simulink model "Torre"  (R2023a)
settings: Solver=VariableStepAuto  StartTime=0.0  StopTime=10  RelTol=1e-3
values from neighbouring files (symbols this model uses):
  a = 5.68    [setup.m]    (also in setup_simple.m)
  B = 14.32    [setup.m]    (also in setup_simple.m)
  D = 8.7775    [setup.m]    (also in setup_simple.m)
  L = 7.3916    [setup.m]    (also in setup_simple.m)
  Lf = 13.3973    [setup.m]    (also in setup_simple.m)
  M = 5.80    (= 5.8)    [setup.m]    (also in setup_simple.m)
  Mb = 31.11    [setup.m]    (also in setup_simple.m)
  Md = 13.07    [setup.m]    (also in setup_simple.m)
  V = 6.4677    [setup.m]    (also in setup_simple.m)
  Vf = 9.7015    [setup.m]    (also in setup_simple.m)
  XF = 0.26095    [setup.m]    (also in setup_simple.m)
  YF = 0.66728    [setup.m]    (also in setup_simple.m)
libraries: slpidlib x2
settings Model: Creator=11106979966  LastModifiedBy=pedro
settings SolverCC: ZeroCrossAlgorithm=Adaptive  AlgebraicLoopSolver=TrustRegion
settings DataIOCC: ReturnWorkspaceOutputs=off
settings DebuggingCC: IgnoredZcDiagnostic=none  UnconnectedInputMsg=warning  UnconnectedOutputMsg=warning  UnconnectedLineMsg=warning  ArithmeticOperatorsInVariantConditions=warning
settings ModelReferenceCC: EnableRefExpFcnMdlSchedulingChecks=on
settings SFSimCC: SimUseLocalCustomCode=off  CustomCodeUndefinedFunction=UseInterfaceOnly
settings RTWCC: RTWUseLocalCustomCode=off
settings CodeAppCC: StateflowObjectComments=on

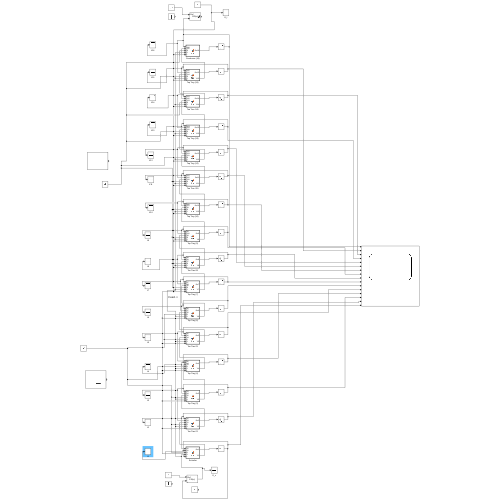
[thumbnail: Simulink's stored preview of the top-level diagram]
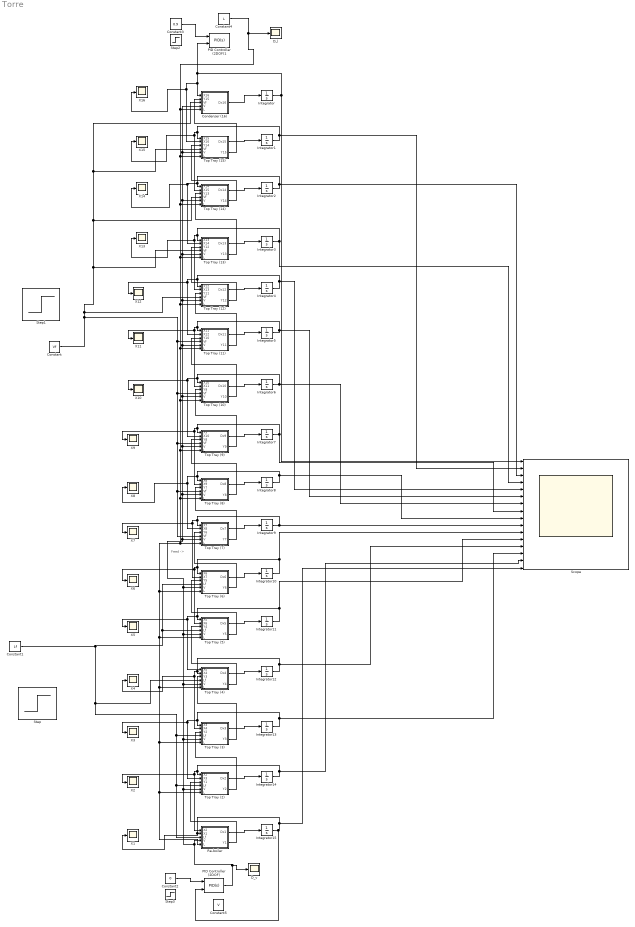
== system Torre ==
  note: Feed ->
  "Condenser (16) " : MATLAB Function  TreatAsAtomicUnit=on
  Constant : Constant  Value=Vf
  Constant1 : Constant  Value=Lf
  Constant2 : Constant  Value=0
  Constant3 : Constant  Value=0.9
  Constant4 : Constant  Value=L
  Constant5 : Constant  Value=V
  D_l : Scope
  D_v : Scope
  Integrator{,1..15} (16 alike) : Integrator  LimitOutput=on  UpperSaturationLimit=1  LowerSaturationLimit=0
  PID Controller (2DOF) : slpidlib/PID Controller (2DOF)  Controller=PID  Form=Parallel  TimeDomain=Continuous-time  UseExternalTs=off  SampleTime=-1  IntegratorMethod=Forward Euler  FilterMethod=Forward Euler  ControllerParametersSource=internal  P=-10000  I=0  UseKiTs=off  D=0  N=100  UseFilter=on  b=1  c=1  TunerSelectOption=Transfer Function Based (PID Tuner App)  InitialConditionSource=internal  InitialConditionForIntegrator=0  InitialConditionForFilter=0  DifferentiatorICPrevScaledInput=0  ExternalReset=none  TrackingMode=off  Kt=1  LimitOutput=off  SatLimitsSource=internal  UpperSaturationLimit=inf  LowerSaturationLimit=-inf  LinearizeAsGain=on  AntiWindupMode=none  Kb=1  LimitIntegrator=off  UpperIntegratorSaturationLimit=inf  LowerIntegratorSaturationLimit=-inf  POutMin=[]  POutMax=[]  IOutMin=[]  IOutMax=[]  DOutMin=[]  DOutMax=[]  NOutMin=[]  NOutMax=[]  bOutMin=[]  bOutMax=[]  cOutMin=[]  cOutMax=[]  SumOutMin=[]  SumOutMax=[]  SaturationOutMin=[]  SaturationOutMax=[]  PParamMin=[]  PParamMax=[]  IParamMin=[]  IParamMax=[]  DParamMin=[]  DParamMax=[]  NParamMin=[]  NParamMax=[]  bParamMin=[]  bParamMax=[]  cParamMin=[]  cParamMax=[]  KbParamMin=[]  KbParamMax=[]  KtParamMin=[]  KtParamMax=[]  KbOutMin=[]  KbOutMax=[]  KtOutMin=[]  KtOutMax=[]  IntegratorOutMin=[]  IntegratorOutMax=[]  FilterOutMin=[]  FilterOutMax=[]  SumI1OutMin=[]  SumI1OutMax=[]  SumI2OutMin=[]  SumI2OutMax=[]  SumI3OutMin=[]  SumI3OutMax=[]  SumI4OutMin=[]  SumI4OutMax=[]  SumDOutMin=[]  SumDOutMax=[]  Sum1OutMin=[]  Sum1OutMax=[]  Sum2OutMin=[]  Sum2OutMax=[]  Sum3OutMin=[]  Sum3OutMax=[]  DifferentiatorOutMin=[]  DifferentiatorOutMax=[]  FilterDiffOutCoefMin=[]  FilterDiffOutCoefMax=[]  ReciprocalOutMin=[]  ReciprocalOutMax=[]  SumDenOutMin=[]  SumDenOutMax=[]  SumNumOutMin=[]  SumNumOutMax=[]  DivideOutMin=[]  DivideOutMax=[]  UdiffTsProdOutMin=[]  UdiffTsProdOutMax=[]  NTsProdOutMin=[]  NTsProdOutMax=[]  UintegralTsProdOutMin=[]  UintegralTsProdOutMax=[]  UngainTsProdOutMin=[]  UngainTsProdOutMax=[]  ClampingZeroOutDataTypeStr=Inherit: Inherit via back propagation  ClampingZeroOutMin=[]  ClampingZeroOutMax=[]  FilterDenConstantOutDataTypeStr=Inherit: Inherit via back propagation  FilterDenConstantOutMin=[]  FilterDenConstantOutMax=[]  PCopyOutDataTypeStr=Inherit: Inherit via back propagation  PCopyOutMin=[]  PCopyOutMax=[]  NCopyOutDataTypeStr=Inherit: Inherit via back propagation  NCopyOutMin=[]  NCopyOutMax=[]  IntegratorContinuousStateAttributes=''  IntegratorStateMustResolveToSignalObject=off  IntegratorRTWStateStorageClass=Auto  FilterContinuousStateAttributes=''  FilterStateMustResolveToSignalObject=off  FilterRTWStateStorageClass=Auto  ParallelPVariant=InternalParameters  IdealPVariant=Disabled  IVariant=InternalParameters  DVariant=InternalParameters  bVariant=InternalParameters  cVariant=InternalParameters  IntegratorVariant=Continuous  SatVariant=Disabled  AWVariant=Passthrough  PCopyVariant=Disabled  TRVariant=Disabled  FdbkBlocksVariant=Forward  IdealPFdbkVariant=Disabled  SatFdbkVariant=Disabled  DerivativeFilterVariant=ContFilter  NVariant=InternalParameters  NCopyVariant=Disabled  FilterICVariant=InternalICsFilter  IntegratorICVariant=InternalICs  ExternalResetVariant=Disabled  TRSumVariant=Passthrough  SumFdbkVariant=Disabled  SumVariant=Sum_PID  TsampFilterVariant=InternalTs  TsampNgainVariant=Passthrough  TsampIntegralVariant=Disabled_SignalSpec  ExternalSaturationOutDataTypeStr=Inherit: Same as second input
  PID Controller (2DOF)1 : slpidlib/PID Controller (2DOF)  Controller=PID  Form=Parallel  TimeDomain=Continuous-time  UseExternalTs=off  SampleTime=-1  IntegratorMethod=Forward Euler  FilterMethod=Forward Euler  ControllerParametersSource=internal  P=-1000  I=0  UseKiTs=off  D=0.7  N=100  UseFilter=on  b=1  c=1  TunerSelectOption=Transfer Function Based (PID Tuner App)  InitialConditionSource=internal  InitialConditionForIntegrator=0  InitialConditionForFilter=0  DifferentiatorICPrevScaledInput=0  ExternalReset=none  TrackingMode=off  Kt=1  LimitOutput=on  SatLimitsSource=internal  UpperSaturationLimit=inf  LowerSaturationLimit=0  LinearizeAsGain=on  AntiWindupMode=none  Kb=1  LimitIntegrator=off  UpperIntegratorSaturationLimit=inf  LowerIntegratorSaturationLimit=-inf  POutMin=[]  POutMax=[]  IOutMin=[]  IOutMax=[]  DOutMin=[]  DOutMax=[]  NOutMin=[]  NOutMax=[]  bOutMin=[]  bOutMax=[]  cOutMin=[]  cOutMax=[]  SumOutMin=[]  SumOutMax=[]  SaturationOutMin=[]  SaturationOutMax=[]  PParamMin=[]  PParamMax=[]  IParamMin=[]  IParamMax=[]  DParamMin=[]  DParamMax=[]  NParamMin=[]  NParamMax=[]  bParamMin=[]  bParamMax=[]  cParamMin=[]  cParamMax=[]  KbParamMin=[]  KbParamMax=[]  KtParamMin=[]  KtParamMax=[]  KbOutMin=[]  KbOutMax=[]  KtOutMin=[]  KtOutMax=[]  IntegratorOutMin=[]  IntegratorOutMax=[]  FilterOutMin=[]  FilterOutMax=[]  SumI1OutMin=[]  SumI1OutMax=[]  SumI2OutMin=[]  SumI2OutMax=[]  SumI3OutMin=[]  SumI3OutMax=[]  SumI4OutMin=[]  SumI4OutMax=[]  SumDOutMin=[]  SumDOutMax=[]  Sum1OutMin=[]  Sum1OutMax=[]  Sum2OutMin=[]  Sum2OutMax=[]  Sum3OutMin=[]  Sum3OutMax=[]  DifferentiatorOutMin=[]  DifferentiatorOutMax=[]  FilterDiffOutCoefMin=[]  FilterDiffOutCoefMax=[]  ReciprocalOutMin=[]  ReciprocalOutMax=[]  SumDenOutMin=[]  SumDenOutMax=[]  SumNumOutMin=[]  SumNumOutMax=[]  DivideOutMin=[]  DivideOutMax=[]  UdiffTsProdOutMin=[]  UdiffTsProdOutMax=[]  NTsProdOutMin=[]  NTsProdOutMax=[]  UintegralTsProdOutMin=[]  UintegralTsProdOutMax=[]  UngainTsProdOutMin=[]  UngainTsProdOutMax=[]  ClampingZeroOutDataTypeStr=Inherit: Inherit via back propagation  ClampingZeroOutMin=[]  ClampingZeroOutMax=[]  FilterDenConstantOutDataTypeStr=Inherit: Inherit via back propagation  FilterDenConstantOutMin=[]  FilterDenConstantOutMax=[]  PCopyOutDataTypeStr=Inherit: Inherit via back propagation  PCopyOutMin=[]  PCopyOutMax=[]  NCopyOutDataTypeStr=Inherit: Inherit via back propagation  NCopyOutMin=[]  NCopyOutMax=[]  IntegratorContinuousStateAttributes=''  IntegratorStateMustResolveToSignalObject=off  IntegratorRTWStateStorageClass=Auto  FilterContinuousStateAttributes=''  FilterStateMustResolveToSignalObject=off  FilterRTWStateStorageClass=Auto  ParallelPVariant=InternalParameters  IdealPVariant=Disabled  IVariant=InternalParameters  DVariant=InternalParameters  bVariant=InternalParameters  cVariant=InternalParameters  IntegratorVariant=Continuous  SatVariant=Enabled  AWVariant=Passthrough  PCopyVariant=Disabled  TRVariant=Disabled  FdbkBlocksVariant=Forward  IdealPFdbkVariant=Disabled  SatFdbkVariant=Disabled  DerivativeFilterVariant=ContFilter  NVariant=InternalParameters  NCopyVariant=Disabled  FilterICVariant=InternalICsFilter  IntegratorICVariant=InternalICs  ExternalResetVariant=Disabled  TRSumVariant=Passthrough  SumFdbkVariant=Disabled  SumVariant=Sum_PID  TsampFilterVariant=InternalTs  TsampNgainVariant=Passthrough  TsampIntegralVariant=Disabled_SignalSpec  ExternalSaturationOutDataTypeStr=Inherit: Same as second input
  Re-boiler : MATLAB Function  TreatAsAtomicUnit=on
  Scope : Scope  NumInputPorts=16
  Step : Step  Time=150  Before=13.3973  After=8.5  SampleTime=0
  Step1 : Step  Time=150  Before=9.7015  After=15.6258  SampleTime=0
  Step2 : Step  Time=20  Before=0.8  SampleTime=0
  Step3 : Step  Time=50  After=0.1  SampleTime=0
  Top Tray (10) : MATLAB Function  TreatAsAtomicUnit=on
  Top Tray (11) : MATLAB Function  TreatAsAtomicUnit=on
  Top Tray (12) : MATLAB Function  TreatAsAtomicUnit=on
  Top Tray (13) : MATLAB Function  TreatAsAtomicUnit=on
  Top Tray (14) : MATLAB Function  TreatAsAtomicUnit=on
  Top Tray (15) : MATLAB Function  TreatAsAtomicUnit=on
  Top Tray (2) : MATLAB Function  TreatAsAtomicUnit=on
  Top Tray (3) : MATLAB Function  TreatAsAtomicUnit=on
  Top Tray (4) : MATLAB Function  TreatAsAtomicUnit=on
  Top Tray (5) : MATLAB Function  TreatAsAtomicUnit=on
  Top Tray (6) : MATLAB Function  TreatAsAtomicUnit=on
  Top Tray (7) : MATLAB Function  TreatAsAtomicUnit=on
  Top Tray (8) : MATLAB Function  TreatAsAtomicUnit=on
  Top Tray (9) : MATLAB Function  TreatAsAtomicUnit=on
  X{1..12} (12 alike) : Scope
  "X13 " : Scope
  "X14 " : Scope
  "X15 " : Scope
  "X16 " : Scope
  wires:
  "Condenser (16) "/1(Dx16) -> Integrator/1
  Integrator/1 -> PID Controller (2DOF)1/2, "X16 "/1, Top Tray (15)/2(X16), "Condenser (16) "/1(X16), Scope/1
  Top Tray (15)/1(Dx15) -> Integrator1/1
  Top Tray (14)/1(Dx14) -> Integrator2/1
  Integrator2/1 -> "X14 "/1, Top Tray (13)/2(X14), Top Tray (14)/1(X14), Scope/3
  Top Tray (13)/1(Dx13) -> Integrator3/1
  Integrator3/1 -> "X13 "/1, Top Tray (12)/2(X13), Top Tray (13)/1(X13), Scope/4
  Integrator4/1 -> Scope/5, X12/1, Top Tray (11)/2(X12), Top Tray (12)/1(X12)
  Top Tray (12)/1(Dx12) -> Integrator4/1
  Integrator5/1 -> X11/1, Top Tray (10)/2(X11), Top Tray (11)/1(X11), Scope/6
  Top Tray (11)/1(Dx11) -> Integrator5/1
  Integrator6/1 -> Top Tray (9)/2(X10), X10/1, Top Tray (10)/1(X10), Scope/7
  Top Tray (10)/1(Dx10) -> Integrator6/1
  Top Tray (9)/1(Dx9) -> Integrator7/1
  Integrator7/1 -> X9/1, Top Tray (8)/2(X9), Top Tray (9)/1(X9), Scope/8
  Integrator8/1 -> Scope/9, X8/1, Top Tray (7)/2(X8), Top Tray (8)/1(X8)
  Top Tray (8)/1(Dx8) -> Integrator8/1
  Integrator9/1 -> X7/1, Top Tray (6)/2(X7), Top Tray (7)/1(X7), Scope/10
  Top Tray (7)/1(Dx7) -> Integrator9/1
  Top Tray (6)/1(Dx6) -> Integrator10/1
  Top Tray (5)/1(Dx5) -> Integrator11/1
  Top Tray (4)/1(Dx4) -> Integrator12/1
  Integrator12/1 -> Scope/13, X4/1, Top Tray (3)/2(X4), Top Tray (4)/2(X4)
  Top Tray (3)/1(Dx3) -> Integrator13/1
  Integrator13/1 -> Scope/14, X3/1, Top Tray (2)/2(X3), Top Tray (3)/1(X3)
  Top Tray (2)/1(Dx2) -> Integrator14/1
  Integrator14/1 -> Scope/15, X2/1, Re-boiler/1(X2), Top Tray (2)/1(X2)
  Re-boiler/1(Dx1) -> Integrator15/1
  Top Tray (15)/2(Y15) -> "Condenser (16) "/2(Y15)
  Top Tray (14)/2(Y14) -> Top Tray (15)/3(Y14)
  Integrator1/1 -> "X15 "/1, Top Tray (14)/2(X15), Top Tray (15)/1(X15), Scope/2
  Top Tray (13)/2(Y13) -> Top Tray (14)/3(Y13)
  Top Tray (12)/2(Y12) -> Top Tray (13)/3(Y12)
  Top Tray (11)/2(Y11) -> Top Tray (12)/3(Y11)
  Top Tray (10)/2(Y10) -> Top Tray (11)/3(Y10)
  Top Tray (9)/2(Y9) -> Top Tray (10)/3(Y9)
  Top Tray (8)/2(Y8) -> Top Tray (9)/3(Y8)
  Top Tray (7)/2(Y7) -> Top Tray (8)/3(Y7)
  Top Tray (6)/2(Y6) -> Top Tray (7)/3(Y6)
  Top Tray (5)/2(Y5) -> Top Tray (6)/3(Y5)
  Top Tray (4)/2(Y4) -> Top Tray (5)/3(Y4)
  Top Tray (3)/2(Y3) -> Top Tray (4)/3(Y3)
  Top Tray (2)/2(Y2) -> Top Tray (3)/3(Y2)
  Re-boiler/2(Y1) -> Top Tray (2)/3(Y1)
  Integrator10/1 -> Scope/11, X6/1, Top Tray (5)/2(X6), Top Tray (6)/1(X6)
  Integrator11/1 -> Scope/12, X5/1, Top Tray (4)/1(X5), Top Tray (5)/1(X5)
  Constant1/1 -> Re-boiler/3(Lf), Top Tray (2)/4(Lf), Top Tray (3)/4(Lf), Top Tray (4)/4(Lf), Top Tray (6)/4(Lf), Top Tray (5)/4(Lf)
  Constant/1 -> Top Tray (13)/4(Vf), Top Tray (14)/4(Vf), Top Tray (15)/4(Vf), "Condenser (16) "/3(Vf), Top Tray (12)/4(Vf), Top Tray (7)/4(Vf), Top Tray (8)/4(Vf), Top Tray (9)/4(Vf), Top Tray (10)/4(Vf), Top Tray (11)/4(Vf)
  Integrator15/1 -> PID Controller (2DOF)/2, Scope/16, X1/1, Re-boiler/2(X1)
  Constant2/1 -> PID Controller (2DOF)/1
  PID Controller (2DOF)/1 -> D_v/1, "Condenser (16) "/4(V), Top Tray (15)/5(V), Top Tray (14)/5(V), Top Tray (13)/5(V), Top Tray (12)/5(V), Top Tray (11)/5(V), Top Tray (10)/5(V), Top Tray (9)/5(V), Top Tray (8)/5(V), Top Tray (7)/5(V), Top Tray (6)/5(V), Top Tray (5)/5(V), Top Tray (4)/5(V), Top Tray (3)/5(V), Top Tray (2)/5(V), Re-boiler/4(V)
  Constant3/1 -> PID Controller (2DOF)1/1
  Constant4/1 -> Re-boiler/5(L), Top Tray (2)/6(L), Top Tray (3)/6(L), Top Tray (4)/6(L), Top Tray (5)/6(L), Top Tray (6)/6(L), Top Tray (7)/6(L), Top Tray (8)/6(L), Top Tray (9)/6(L), Top Tray (10)/6(L), Top Tray (11)/6(L), Top Tray (12)/6(L), Top Tray (13)/6(L), Top Tray (14)/6(L), Top Tray (15)/6(L), "Condenser (16) "/5(L), D_l/1

== matlab function Torre/Top Tray (9) ==
  data: X9 input; X10 input; Dx9 output; Y8 input; Y9 output; a parameter; M parameter; Vf input; V input; L input
function [Dx9,Y9] = fcn(X9,X10, Y8, a, M, Vf, V, L)

Y9 = (a * X9)/(1+(a-1)*X9);

Dx9 = ((V+Vf)*(Y8-Y9) + L*(X10-X9))/(M);

== matlab function Torre/Top Tray (8) ==
  data: X8 input; X9 input; Dx8 output; Y7 input; Y8 output; a parameter; M parameter; Vf input; V input; L input
function [Dx8,Y8] = fcn(X8,X9,Y7, a, M, Vf, V, L)

Y8 = (a * X8)/(1+(a-1)*X8);

Dx8 = ((V+Vf)*(Y7-Y8) + L*(X9-X8))/(M);

== matlab function Torre/Top Tray (7) ==
  data: X7 input; X8 input; Y6 input; Dx7 output; Y7 output; a parameter; M parameter; YF parameter; Vf input; V input; L input
function [Dx7,Y7] = fcn(X7,X8, Y6, a, M, YF, Vf, V, L)

Y7 = (a * X7)/(1+(a-1)*X7);

Dx7 = (V*(Y6-Y7) + L*(X8-X7) + Vf*(YF-Y7))/(M);

== matlab function Torre/Top Tray (6) ==
  data: X6 input; X7 input; Y5 input; Dx6 output; Y6 output; a parameter; M parameter; XF parameter; Lf input; V input; L input
function [Dx6,Y6] = fcn(X6,X7,Y5, a, M, XF, Lf, V, L)

Y6 = (a * X6)/(1+(a-1)*X6);

Dx6 = (V*(Y5-Y6) + L*(X7-X6) + Lf*(XF-X6))/(M);

== matlab function Torre/Top Tray (5) ==
  data: X5 input; X6 input; Y4 input; Dx5 output; Y5 output; a parameter; M parameter; Lf input; V input; L input
function [Dx5,Y5] = fcn(X5,X6, Y4, a, M, Lf, V, L)

Y5 = (a * X5)/(1+(a-1)*X5);

Dx5 = (V*(Y4-Y5) + (L+Lf)*(X6-X5))/(M);

== matlab function Torre/Top Tray (14) ==
  data: X14 input; X15 input; Dx14 output; Y13 input; Y14 output; a parameter; M parameter; Vf input; V input; L input
function [Dx14,Y14] = fcn(X14,X15, Y13, a, M, Vf, V, L)

Y14 = (a * X14)/(1+(a-1)*X14);

Dx14 = ((V+Vf)*(Y13-Y14) + L*(X15-X14))/(M);

== matlab function Torre/Top Tray (4) ==
  data: X5 input; X4 input; Y3 input; Dx4 output; Y4 output; a parameter; M parameter; Lf input; V input; L input
function [Dx4,Y4] = fcn(X5,X4, Y3, a, M, Lf, V, L)

Y4 = (a * X4)/(1+(a-1)*X4);

Dx4 = (V*(Y3-Y4) + (L+Lf)*(X5-X4))/(M);

== matlab function Torre/Top Tray (3) ==
  data: X3 input; X4 input; Y2 input; Dx3 output; Y3 output; a parameter; M parameter; Lf input; V input; L input
function [Dx3,Y3] = fcn(X3,X4, Y2, a, M, Lf, V, L)

Y3 = (a * X3)/(1+(a-1)*X3);

Dx3 = (V*(Y2-Y3) + (L+Lf)*(X4-X3))/(M);

== matlab function Torre/Top Tray (2) ==
  data: X2 input; X3 input; Y1 input; Dx2 output; Y2 output; a parameter; M parameter; Lf input; V input; L input
function [Dx2,Y2] = fcn(X2,X3, Y1, a, M, Lf, V, L)

Y2 = (a * X2)/(1+(a-1)*X2);

Dx2 = (V*(Y1-Y2) + (L+Lf)*(X3-X2))/(M);

== matlab function Torre/Condenser (16)  ==
  data: Dx16 output; X16 input; Md parameter; D parameter; Y15 input; Vf input; V input; L input
function Dx16  = fcn(X16, Md, D, Y15, Vf, V, L)


Dx16 = ((V + Vf)*Y15 - L*X16 - D*X16)/(Md);

== matlab function Torre/Re-boiler ==
  data: X2 input; X1 input; a parameter; Mb parameter; Dx1 output; Y1 output; B parameter; Lf input; V input; L input
function [Dx1,Y1] = fcn(X2,X1, a, Mb, B, Lf, V, L)

Y1 = (a * X1)/(1+(a-1)*X1);

Dx1 = ((L+Lf)*(X2) -V*Y1 -B*X1 )/(Mb);

== matlab function Torre/Top Tray (15) ==
  data: X15 input; X16 input; Dx15 output; Y14 input; Y15 output; a parameter; M parameter; Vf input; V input; L input
function [Dx15,Y15] = fcn(X15,X16,Y14, a, M, Vf, V, L)

Y15 = (a * X15)/(1+(a-1)*X15);

Dx15 = ((V+Vf)*(Y14-Y15) + L*(X16-X15))/(M);

== matlab function Torre/Top Tray (13) ==
  data: X13 input; X14 input; Dx13 output; Y12 input; Y13 output; a parameter; M parameter; Vf input; V input; L input
function [Dx13,Y13] = fcn(X13,X14, Y12, a, M, Vf, V, L)

Y13 = (a * X13)/(1+(a-1)*X13);

Dx13 = ((V+Vf)*(Y12-Y13) + L*(X14-X13))/(M);

== matlab function Torre/Top Tray (12) ==
  data: X12 input; X13 input; Dx12 output; Y11 input; Y12 output; a parameter; M parameter; Vf input; V input; L input
function [Dx12,Y12] = fcn(X12,X13, Y11, a, M, Vf, V, L)

Y12 = (a * X12)/(1+(a-1)*X12);

Dx12 = ((V+Vf)*(Y11-Y12) + L*(X13-X12))/(M);

== matlab function Torre/Top Tray (11) ==
  data: X11 input; X12 input; Dx11 output; Y10 input; Y11 output; a parameter; M parameter; Vf input; V input; L input
function [Dx11,Y11] = fcn(X11,X12, Y10, a, M, Vf, V, L)

Y11 = (a * X11)/(1+(a-1)*X11);

Dx11 = ((V+Vf)*(Y10-Y11) + L*(X12-X11))/(M);

== matlab function Torre/Top Tray (10) ==
  data: X10 input; X11 input; Dx10 output; Y9 input; Y10 output; a parameter; M parameter; Vf input; V input; L input
function [Dx10,Y10] = fcn(X10,X11, Y9, a, M, Vf, V, L)

Y10 = (a * X10)/(1+(a-1)*X10);

Dx10 = ((V+Vf)*(Y9-Y10) + L*(X11-X10))/(M);
